simulink model "CM475A_TSG31CfgAndUse"  (R2013b)
settings: Solver=FixedStepDiscrete  SolverMode=SingleTasking  StartTime=0.0  StopTime=0.5  FixedStep=0.00005  RelTol=1e-3
undefined symbols (not defined in the file): ELECGLBPRM_PWMPERDMIN_NANOSEC_U32, sigbuilder_block, SysSt1, TSG31CfgAndUseAdcStrtOfCnvn2Offs, TSG31CfgAndUseAdcStrtOfCnvnMotCtrlPeakOffs, TSG31CfgAndUseAdcStrtOfCnvnMotCtrlVlyOffs, TSG31CfgAndUseMtrAg0SPIStart, TSG31CfgAndUsePwmDbnd, TSG31UPD_NANOSEC_U32
libraries: simulink x11, CM475A_TSG31CfgAndUse_ModelLibrary_Rev001 x11
(part 4 of 4)

== system CM475A_TSG31CfgAndUse/TSG31CfgAndUse/TSG31CfgAndUsePer2/No Transition SysState = Enable/MCECS_OFFSCMDEND and MCECS_GAINCMDAD/Map Pins to GPIO/IoHwAb_SetFctGpioPhaALowrCmd ==
  CopyRight2 : Subsystem  Description=|  mask(Copyright Information){none=on}
      | Copyright info block.                                               
      |                                                                     
      | Place copyright information at the top of every subsystem in design.
      mask prompts: none "No parameters"
      mask help: Place copyright information at the top of every subsystem in design.
      mask Display:
      | NxtrConf = 'Nexteer Confidential';
      | 
      | sys = bdroot; %handle for the current model ("system")
      | first = get_param(sys,'Created');
      | first = first(end-3:end);  %year is last four digits
      | 
      | last = get_param(sys,'LastModifiedDate');
      | if isempty(last)
      |     last = datestr(now,'yyyy');
      | else
      |     last = last(end-3:end);
      | end
      | 
      | if strcmp(first,last)
      |     fprintf('%s -- Copyright %s Nexteer',NxtrConf,first)
      | else
      |     fprintf('%s -- %s%s- %s Nexteer',NxtrConf,char(169),first,last)
      | end

== system CM475A_TSG31CfgAndUse/TSG31CfgAndUse/TSG31CfgAndUsePer2/No Transition SysState = Enable/MCECS_OFFSCMDEND and MCECS_GAINCMDAD/Map Pins to GPIO/IoHwAb_SetFctGpioPhaAUpprCmd ==
  CopyRight2 : Subsystem  Description=|  mask(Copyright Information){none=on}
      | Copyright info block.                                               
      |                                                                     
      | Place copyright information at the top of every subsystem in design.
      mask prompts: none "No parameters"
      mask help: Place copyright information at the top of every subsystem in design.
      mask Display:
      | NxtrConf = 'Nexteer Confidential';
      | 
      | sys = bdroot; %handle for the current model ("system")
      | first = get_param(sys,'Created');
      | first = first(end-3:end);  %year is last four digits
      | 
      | last = get_param(sys,'LastModifiedDate');
      | if isempty(last)
      |     last = datestr(now,'yyyy');
      | else
      |     last = last(end-3:end);
      | end
      | 
      | if strcmp(first,last)
      |     fprintf('%s -- Copyright %s Nexteer',NxtrConf,first)
      | else
      |     fprintf('%s -- %s%s- %s Nexteer',NxtrConf,char(169),first,last)
      | end

== system CM475A_TSG31CfgAndUse/TSG31CfgAndUse/TSG31CfgAndUsePer2/No Transition SysState = Enable/MCECS_OFFSCMDEND and MCECS_GAINCMDAD/Map Pins to GPIO/IoHwAb_SetFctGpioPhaBLowrCmd ==
  CopyRight2 : Subsystem  Description=|  mask(Copyright Information){none=on}
      | Copyright info block.                                               
      |                                                                     
      | Place copyright information at the top of every subsystem in design.
      mask prompts: none "No parameters"
      mask help: Place copyright information at the top of every subsystem in design.
      mask Display:
      | NxtrConf = 'Nexteer Confidential';
      | 
      | sys = bdroot; %handle for the current model ("system")
      | first = get_param(sys,'Created');
      | first = first(end-3:end);  %year is last four digits
      | 
      | last = get_param(sys,'LastModifiedDate');
      | if isempty(last)
      |     last = datestr(now,'yyyy');
      | else
      |     last = last(end-3:end);
      | end
      | 
      | if strcmp(first,last)
      |     fprintf('%s -- Copyright %s Nexteer',NxtrConf,first)
      | else
      |     fprintf('%s -- %s%s- %s Nexteer',NxtrConf,char(169),first,last)
      | end

== system CM475A_TSG31CfgAndUse/TSG31CfgAndUse/TSG31CfgAndUsePer2/No Transition SysState = Enable/MCECS_OFFSCMDEND and MCECS_GAINCMDAD/Map Pins to GPIO/IoHwAb_SetFctGpioPhaBUpprCmd ==
  CopyRight2 : Subsystem  Description=|  mask(Copyright Information){none=on}
      | Copyright info block.                                               
      |                                                                     
      | Place copyright information at the top of every subsystem in design.
      mask prompts: none "No parameters"
      mask help: Place copyright information at the top of every subsystem in design.
      mask Display:
      | NxtrConf = 'Nexteer Confidential';
      | 
      | sys = bdroot; %handle for the current model ("system")
      | first = get_param(sys,'Created');
      | first = first(end-3:end);  %year is last four digits
      | 
      | last = get_param(sys,'LastModifiedDate');
      | if isempty(last)
      |     last = datestr(now,'yyyy');
      | else
      |     last = last(end-3:end);
      | end
      | 
      | if strcmp(first,last)
      |     fprintf('%s -- Copyright %s Nexteer',NxtrConf,first)
      | else
      |     fprintf('%s -- %s%s- %s Nexteer',NxtrConf,char(169),first,last)
      | end

== system CM475A_TSG31CfgAndUse/TSG31CfgAndUse/TSG31CfgAndUsePer2/No Transition SysState = Enable/MCECS_OFFSCMDEND and MCECS_GAINCMDAD/Map Pins to GPIO/IoHwAb_SetFctGpioPhaCLowrCmd ==
  CopyRight2 : Subsystem  Description=|  mask(Copyright Information){none=on}
      | Copyright info block.                                               
      |                                                                     
      | Place copyright information at the top of every subsystem in design.
      mask prompts: none "No parameters"
      mask help: Place copyright information at the top of every subsystem in design.
      mask Display:
      | NxtrConf = 'Nexteer Confidential';
      | 
      | sys = bdroot; %handle for the current model ("system")
      | first = get_param(sys,'Created');
      | first = first(end-3:end);  %year is last four digits
      | 
      | last = get_param(sys,'LastModifiedDate');
      | if isempty(last)
      |     last = datestr(now,'yyyy');
      | else
      |     last = last(end-3:end);
      | end
      | 
      | if strcmp(first,last)
      |     fprintf('%s -- Copyright %s Nexteer',NxtrConf,first)
      | else
      |     fprintf('%s -- %s%s- %s Nexteer',NxtrConf,char(169),first,last)
      | end

== system CM475A_TSG31CfgAndUse/TSG31CfgAndUse/TSG31CfgAndUsePer2/No Transition SysState = Enable/MCECS_OFFSCMDEND and MCECS_GAINCMDAD/Map Pins to GPIO/IoHwAb_SetFctGpioPhaCUpprCmd ==
  CopyRight2 : Subsystem  Description=|  mask(Copyright Information){none=on}
      | Copyright info block.                                               
      |                                                                     
      | Place copyright information at the top of every subsystem in design.
      mask prompts: none "No parameters"
      mask help: Place copyright information at the top of every subsystem in design.
      mask Display:
      | NxtrConf = 'Nexteer Confidential';
      | 
      | sys = bdroot; %handle for the current model ("system")
      | first = get_param(sys,'Created');
      | first = first(end-3:end);  %year is last four digits
      | 
      | last = get_param(sys,'LastModifiedDate');
      | if isempty(last)
      |     last = datestr(now,'yyyy');
      | else
      |     last = last(end-3:end);
      | end
      | 
      | if strcmp(first,last)
      |     fprintf('%s -- Copyright %s Nexteer',NxtrConf,first)
      | else
      |     fprintf('%s -- %s%s- %s Nexteer',NxtrConf,char(169),first,last)
      | end

== system CM475A_TSG31CfgAndUse/TSG31CfgAndUse/TSG31CfgAndUsePer2/No Transition SysState = Enable/MCECS_OFFSCMDEND and MCECS_GAINCMDAD/Set GPIO Level/CopyRight2 ==

== system CM475A_TSG31CfgAndUse/TSG31CfgAndUse/TSG31CfgAndUsePer2/No Transition SysState = Enable/MCECS_OFFSCMDEND and MCECS_GAINCMDAD/Set GPIO Level/IoHwAb_SetGpioPhaALowrCmd ==
  PinSt : Inport  OutDataTypeStr=boolean
  CopyRight2 : Subsystem  Description=|  mask(Copyright Information){none=on}
      | Copyright info block.                                               
      |                                                                     
      | Place copyright information at the top of every subsystem in design.
      mask prompts: none "No parameters"
      mask help: Place copyright information at the top of every subsystem in design.
      mask Display:
      | NxtrConf = 'Nexteer Confidential';
      | 
      | sys = bdroot; %handle for the current model ("system")
      | first = get_param(sys,'Created');
      | first = first(end-3:end);  %year is last four digits
      | 
      | last = get_param(sys,'LastModifiedDate');
      | if isempty(last)
      |     last = datestr(now,'yyyy');
      | else
      |     last = last(end-3:end);
      | end
      | 
      | if strcmp(first,last)
      |     fprintf('%s -- Copyright %s Nexteer',NxtrConf,first)
      | else
      |     fprintf('%s -- %s%s- %s Nexteer',NxtrConf,char(169),first,last)
      | end
  Terminator : Terminator
  wires:
  PinSt/1 -> Terminator/1

== system CM475A_TSG31CfgAndUse/TSG31CfgAndUse/TSG31CfgAndUsePer2/No Transition SysState = Enable/MCECS_OFFSCMDEND and MCECS_GAINCMDAD/Set GPIO Level/IoHwAb_SetGpioPhaAUpprCmd ==
  PinSt : Inport  OutDataTypeStr=boolean
  CopyRight2 : Subsystem  Description=|  mask(Copyright Information){none=on}
      | Copyright info block.                                               
      |                                                                     
      | Place copyright information at the top of every subsystem in design.
      mask prompts: none "No parameters"
      mask help: Place copyright information at the top of every subsystem in design.
      mask Display:
      | NxtrConf = 'Nexteer Confidential';
      | 
      | sys = bdroot; %handle for the current model ("system")
      | first = get_param(sys,'Created');
      | first = first(end-3:end);  %year is last four digits
      | 
      | last = get_param(sys,'LastModifiedDate');
      | if isempty(last)
      |     last = datestr(now,'yyyy');
      | else
      |     last = last(end-3:end);
      | end
      | 
      | if strcmp(first,last)
      |     fprintf('%s -- Copyright %s Nexteer',NxtrConf,first)
      | else
      |     fprintf('%s -- %s%s- %s Nexteer',NxtrConf,char(169),first,last)
      | end
  Terminator : Terminator
  wires:
  PinSt/1 -> Terminator/1

== system CM475A_TSG31CfgAndUse/TSG31CfgAndUse/TSG31CfgAndUsePer2/No Transition SysState = Enable/MCECS_OFFSCMDEND and MCECS_GAINCMDAD/Set GPIO Level/IoHwAb_SetGpioPhaBLowrCmd ==
  PinSt : Inport  OutDataTypeStr=boolean
  CopyRight2 : Subsystem  Description=|  mask(Copyright Information){none=on}
      | Copyright info block.                                               
      |                                                                     
      | Place copyright information at the top of every subsystem in design.
      mask prompts: none "No parameters"
      mask help: Place copyright information at the top of every subsystem in design.
      mask Display:
      | NxtrConf = 'Nexteer Confidential';
      | 
      | sys = bdroot; %handle for the current model ("system")
      | first = get_param(sys,'Created');
      | first = first(end-3:end);  %year is last four digits
      | 
      | last = get_param(sys,'LastModifiedDate');
      | if isempty(last)
      |     last = datestr(now,'yyyy');
      | else
      |     last = last(end-3:end);
      | end
      | 
      | if strcmp(first,last)
      |     fprintf('%s -- Copyright %s Nexteer',NxtrConf,first)
      | else
      |     fprintf('%s -- %s%s- %s Nexteer',NxtrConf,char(169),first,last)
      | end
  Terminator : Terminator
  wires:
  PinSt/1 -> Terminator/1

== system CM475A_TSG31CfgAndUse/TSG31CfgAndUse/TSG31CfgAndUsePer2/No Transition SysState = Enable/MCECS_OFFSCMDEND and MCECS_GAINCMDAD/Set GPIO Level/IoHwAb_SetGpioPhaBUpprCmd ==
  PinSt : Inport  OutDataTypeStr=boolean
  CopyRight2 : Subsystem  Description=|  mask(Copyright Information){none=on}
      | Copyright info block.                                               
      |                                                                     
      | Place copyright information at the top of every subsystem in design.
      mask prompts: none "No parameters"
      mask help: Place copyright information at the top of every subsystem in design.
      mask Display:
      | NxtrConf = 'Nexteer Confidential';
      | 
      | sys = bdroot; %handle for the current model ("system")
      | first = get_param(sys,'Created');
      | first = first(end-3:end);  %year is last four digits
      | 
      | last = get_param(sys,'LastModifiedDate');
      | if isempty(last)
      |     last = datestr(now,'yyyy');
      | else
      |     last = last(end-3:end);
      | end
      | 
      | if strcmp(first,last)
      |     fprintf('%s -- Copyright %s Nexteer',NxtrConf,first)
      | else
      |     fprintf('%s -- %s%s- %s Nexteer',NxtrConf,char(169),first,last)
      | end
  Terminator : Terminator
  wires:
  PinSt/1 -> Terminator/1

== system CM475A_TSG31CfgAndUse/TSG31CfgAndUse/TSG31CfgAndUsePer2/No Transition SysState = Enable/MCECS_OFFSCMDEND and MCECS_GAINCMDAD/Set GPIO Level/IoHwAb_SetGpioPhaCLowrCmd ==
  PinSt : Inport  OutDataTypeStr=boolean
  CopyRight2 : Subsystem  Description=|  mask(Copyright Information){none=on}
      | Copyright info block.                                               
      |                                                                     
      | Place copyright information at the top of every subsystem in design.
      mask prompts: none "No parameters"
      mask help: Place copyright information at the top of every subsystem in design.
      mask Display:
      | NxtrConf = 'Nexteer Confidential';
      | 
      | sys = bdroot; %handle for the current model ("system")
      | first = get_param(sys,'Created');
      | first = first(end-3:end);  %year is last four digits
      | 
      | last = get_param(sys,'LastModifiedDate');
      | if isempty(last)
      |     last = datestr(now,'yyyy');
      | else
      |     last = last(end-3:end);
      | end
      | 
      | if strcmp(first,last)
      |     fprintf('%s -- Copyright %s Nexteer',NxtrConf,first)
      | else
      |     fprintf('%s -- %s%s- %s Nexteer',NxtrConf,char(169),first,last)
      | end
  Terminator : Terminator
  wires:
  PinSt/1 -> Terminator/1

== system CM475A_TSG31CfgAndUse/TSG31CfgAndUse/TSG31CfgAndUsePer2/No Transition SysState = Enable/MCECS_OFFSCMDEND and MCECS_GAINCMDAD/Set GPIO Level/IoHwAb_SetGpioPhaCUpprCmd ==
  PinSt : Inport  OutDataTypeStr=boolean
  CopyRight2 : Subsystem  Description=|  mask(Copyright Information){none=on}
      | Copyright info block.                                               
      |                                                                     
      | Place copyright information at the top of every subsystem in design.
      mask prompts: none "No parameters"
      mask help: Place copyright information at the top of every subsystem in design.
      mask Display:
      | NxtrConf = 'Nexteer Confidential';
      | 
      | sys = bdroot; %handle for the current model ("system")
      | first = get_param(sys,'Created');
      | first = first(end-3:end);  %year is last four digits
      | 
      | last = get_param(sys,'LastModifiedDate');
      | if isempty(last)
      |     last = datestr(now,'yyyy');
      | else
      |     last = last(end-3:end);
      | end
      | 
      | if strcmp(first,last)
      |     fprintf('%s -- Copyright %s Nexteer',NxtrConf,first)
      | else
      |     fprintf('%s -- %s%s- %s Nexteer',NxtrConf,char(169),first,last)
      | end
  Terminator : Terminator
  wires:
  PinSt/1 -> Terminator/1

== system CM475A_TSG31CfgAndUse/TSG31CfgAndUse/TSG31CfgAndUsePer2/Transition from Enable/Map FET Ctrl Signals to GPIO and Set Low/Map Pins to GPIO/CopyRight2 ==

== system CM475A_TSG31CfgAndUse/TSG31CfgAndUse/TSG31CfgAndUsePer2/Transition from Enable/Map FET Ctrl Signals to GPIO and Set Low/Map Pins to GPIO/IoHwAb_SetFctGpioPhaALowrCmd ==
  CopyRight2 : Subsystem  Description=|  mask(Copyright Information){none=on}
      | Copyright info block.                                               
      |                                                                     
      | Place copyright information at the top of every subsystem in design.
      mask prompts: none "No parameters"
      mask help: Place copyright information at the top of every subsystem in design.
      mask Display:
      | NxtrConf = 'Nexteer Confidential';
      | 
      | sys = bdroot; %handle for the current model ("system")
      | first = get_param(sys,'Created');
      | first = first(end-3:end);  %year is last four digits
      | 
      | last = get_param(sys,'LastModifiedDate');
      | if isempty(last)
      |     last = datestr(now,'yyyy');
      | else
      |     last = last(end-3:end);
      | end
      | 
      | if strcmp(first,last)
      |     fprintf('%s -- Copyright %s Nexteer',NxtrConf,first)
      | else
      |     fprintf('%s -- %s%s- %s Nexteer',NxtrConf,char(169),first,last)
      | end

== system CM475A_TSG31CfgAndUse/TSG31CfgAndUse/TSG31CfgAndUsePer2/Transition from Enable/Map FET Ctrl Signals to GPIO and Set Low/Map Pins to GPIO/IoHwAb_SetFctGpioPhaAUpprCmd ==
  CopyRight2 : Subsystem  Description=|  mask(Copyright Information){none=on}
      | Copyright info block.                                               
      |                                                                     
      | Place copyright information at the top of every subsystem in design.
      mask prompts: none "No parameters"
      mask help: Place copyright information at the top of every subsystem in design.
      mask Display:
      | NxtrConf = 'Nexteer Confidential';
      | 
      | sys = bdroot; %handle for the current model ("system")
      | first = get_param(sys,'Created');
      | first = first(end-3:end);  %year is last four digits
      | 
      | last = get_param(sys,'LastModifiedDate');
      | if isempty(last)
      |     last = datestr(now,'yyyy');
      | else
      |     last = last(end-3:end);
      | end
      | 
      | if strcmp(first,last)
      |     fprintf('%s -- Copyright %s Nexteer',NxtrConf,first)
      | else
      |     fprintf('%s -- %s%s- %s Nexteer',NxtrConf,char(169),first,last)
      | end

== system CM475A_TSG31CfgAndUse/TSG31CfgAndUse/TSG31CfgAndUsePer2/Transition from Enable/Map FET Ctrl Signals to GPIO and Set Low/Map Pins to GPIO/IoHwAb_SetFctGpioPhaBLowrCmd ==
  CopyRight2 : Subsystem  Description=|  mask(Copyright Information){none=on}
      | Copyright info block.                                               
      |                                                                     
      | Place copyright information at the top of every subsystem in design.
      mask prompts: none "No parameters"
      mask help: Place copyright information at the top of every subsystem in design.
      mask Display:
      | NxtrConf = 'Nexteer Confidential';
      | 
      | sys = bdroot; %handle for the current model ("system")
      | first = get_param(sys,'Created');
      | first = first(end-3:end);  %year is last four digits
      | 
      | last = get_param(sys,'LastModifiedDate');
      | if isempty(last)
      |     last = datestr(now,'yyyy');
      | else
      |     last = last(end-3:end);
      | end
      | 
      | if strcmp(first,last)
      |     fprintf('%s -- Copyright %s Nexteer',NxtrConf,first)
      | else
      |     fprintf('%s -- %s%s- %s Nexteer',NxtrConf,char(169),first,last)
      | end

== system CM475A_TSG31CfgAndUse/TSG31CfgAndUse/TSG31CfgAndUsePer2/Transition from Enable/Map FET Ctrl Signals to GPIO and Set Low/Map Pins to GPIO/IoHwAb_SetFctGpioPhaBUpprCmd ==
  CopyRight2 : Subsystem  Description=|  mask(Copyright Information){none=on}
      | Copyright info block.                                               
      |                                                                     
      | Place copyright information at the top of every subsystem in design.
      mask prompts: none "No parameters"
      mask help: Place copyright information at the top of every subsystem in design.
      mask Display:
      | NxtrConf = 'Nexteer Confidential';
      | 
      | sys = bdroot; %handle for the current model ("system")
      | first = get_param(sys,'Created');
      | first = first(end-3:end);  %year is last four digits
      | 
      | last = get_param(sys,'LastModifiedDate');
      | if isempty(last)
      |     last = datestr(now,'yyyy');
      | else
      |     last = last(end-3:end);
      | end
      | 
      | if strcmp(first,last)
      |     fprintf('%s -- Copyright %s Nexteer',NxtrConf,first)
      | else
      |     fprintf('%s -- %s%s- %s Nexteer',NxtrConf,char(169),first,last)
      | end

== system CM475A_TSG31CfgAndUse/TSG31CfgAndUse/TSG31CfgAndUsePer2/Transition from Enable/Map FET Ctrl Signals to GPIO and Set Low/Map Pins to GPIO/IoHwAb_SetFctGpioPhaCLowrCmd ==
  CopyRight2 : Subsystem  Description=|  mask(Copyright Information){none=on}
      | Copyright info block.                                               
      |                                                                     
      | Place copyright information at the top of every subsystem in design.
      mask prompts: none "No parameters"
      mask help: Place copyright information at the top of every subsystem in design.
      mask Display:
      | NxtrConf = 'Nexteer Confidential';
      | 
      | sys = bdroot; %handle for the current model ("system")
      | first = get_param(sys,'Created');
      | first = first(end-3:end);  %year is last four digits
      | 
      | last = get_param(sys,'LastModifiedDate');
      | if isempty(last)
      |     last = datestr(now,'yyyy');
      | else
      |     last = last(end-3:end);
      | end
      | 
      | if strcmp(first,last)
      |     fprintf('%s -- Copyright %s Nexteer',NxtrConf,first)
      | else
      |     fprintf('%s -- %s%s- %s Nexteer',NxtrConf,char(169),first,last)
      | end

== system CM475A_TSG31CfgAndUse/TSG31CfgAndUse/TSG31CfgAndUsePer2/Transition from Enable/Map FET Ctrl Signals to GPIO and Set Low/Map Pins to GPIO/IoHwAb_SetFctGpioPhaCUpprCmd ==
  CopyRight2 : Subsystem  Description=|  mask(Copyright Information){none=on}
      | Copyright info block.                                               
      |                                                                     
      | Place copyright information at the top of every subsystem in design.
      mask prompts: none "No parameters"
      mask help: Place copyright information at the top of every subsystem in design.
      mask Display:
      | NxtrConf = 'Nexteer Confidential';
      | 
      | sys = bdroot; %handle for the current model ("system")
      | first = get_param(sys,'Created');
      | first = first(end-3:end);  %year is last four digits
      | 
      | last = get_param(sys,'LastModifiedDate');
      | if isempty(last)
      |     last = datestr(now,'yyyy');
      | else
      |     last = last(end-3:end);
      | end
      | 
      | if strcmp(first,last)
      |     fprintf('%s -- Copyright %s Nexteer',NxtrConf,first)
      | else
      |     fprintf('%s -- %s%s- %s Nexteer',NxtrConf,char(169),first,last)
      | end

== system CM475A_TSG31CfgAndUse/TSG31CfgAndUse/TSG31CfgAndUsePer2/Transition from Enable/Map FET Ctrl Signals to GPIO and Set Low/Set GPIO Level/CopyRight2 ==

== system CM475A_TSG31CfgAndUse/TSG31CfgAndUse/TSG31CfgAndUsePer2/Transition from Enable/Map FET Ctrl Signals to GPIO and Set Low/Set GPIO Level/IoHwAb_SetGpioPhaALowrCmd ==
  PinSt : Inport  OutDataTypeStr=boolean
  CopyRight2 : Subsystem  Description=|  mask(Copyright Information){none=on}
      | Copyright info block.                                               
      |                                                                     
      | Place copyright information at the top of every subsystem in design.
      mask prompts: none "No parameters"
      mask help: Place copyright information at the top of every subsystem in design.
      mask Display:
      | NxtrConf = 'Nexteer Confidential';
      | 
      | sys = bdroot; %handle for the current model ("system")
      | first = get_param(sys,'Created');
      | first = first(end-3:end);  %year is last four digits
      | 
      | last = get_param(sys,'LastModifiedDate');
      | if isempty(last)
      |     last = datestr(now,'yyyy');
      | else
      |     last = last(end-3:end);
      | end
      | 
      | if strcmp(first,last)
      |     fprintf('%s -- Copyright %s Nexteer',NxtrConf,first)
      | else
      |     fprintf('%s -- %s%s- %s Nexteer',NxtrConf,char(169),first,last)
      | end
  Terminator : Terminator
  wires:
  PinSt/1 -> Terminator/1

== system CM475A_TSG31CfgAndUse/TSG31CfgAndUse/TSG31CfgAndUsePer2/Transition from Enable/Map FET Ctrl Signals to GPIO and Set Low/Set GPIO Level/IoHwAb_SetGpioPhaAUpprCmd ==
  PinSt : Inport  OutDataTypeStr=boolean
  CopyRight2 : Subsystem  Description=|  mask(Copyright Information){none=on}
      | Copyright info block.                                               
      |                                                                     
      | Place copyright information at the top of every subsystem in design.
      mask prompts: none "No parameters"
      mask help: Place copyright information at the top of every subsystem in design.
      mask Display:
      | NxtrConf = 'Nexteer Confidential';
      | 
      | sys = bdroot; %handle for the current model ("system")
      | first = get_param(sys,'Created');
      | first = first(end-3:end);  %year is last four digits
      | 
      | last = get_param(sys,'LastModifiedDate');
      | if isempty(last)
      |     last = datestr(now,'yyyy');
      | else
      |     last = last(end-3:end);
      | end
      | 
      | if strcmp(first,last)
      |     fprintf('%s -- Copyright %s Nexteer',NxtrConf,first)
      | else
      |     fprintf('%s -- %s%s- %s Nexteer',NxtrConf,char(169),first,last)
      | end
  Terminator : Terminator
  wires:
  PinSt/1 -> Terminator/1

== system CM475A_TSG31CfgAndUse/TSG31CfgAndUse/TSG31CfgAndUsePer2/Transition from Enable/Map FET Ctrl Signals to GPIO and Set Low/Set GPIO Level/IoHwAb_SetGpioPhaBLowrCmd ==
  PinSt : Inport  OutDataTypeStr=boolean
  CopyRight2 : Subsystem  Description=|  mask(Copyright Information){none=on}
      | Copyright info block.                                               
      |                                                                     
      | Place copyright information at the top of every subsystem in design.
      mask prompts: none "No parameters"
      mask help: Place copyright information at the top of every subsystem in design.
      mask Display:
      | NxtrConf = 'Nexteer Confidential';
      | 
      | sys = bdroot; %handle for the current model ("system")
      | first = get_param(sys,'Created');
      | first = first(end-3:end);  %year is last four digits
      | 
      | last = get_param(sys,'LastModifiedDate');
      | if isempty(last)
      |     last = datestr(now,'yyyy');
      | else
      |     last = last(end-3:end);
      | end
      | 
      | if strcmp(first,last)
      |     fprintf('%s -- Copyright %s Nexteer',NxtrConf,first)
      | else
      |     fprintf('%s -- %s%s- %s Nexteer',NxtrConf,char(169),first,last)
      | end
  Terminator : Terminator
  wires:
  PinSt/1 -> Terminator/1

== system CM475A_TSG31CfgAndUse/TSG31CfgAndUse/TSG31CfgAndUsePer2/Transition from Enable/Map FET Ctrl Signals to GPIO and Set Low/Set GPIO Level/IoHwAb_SetGpioPhaBUpprCmd ==
  PinSt : Inport  OutDataTypeStr=boolean
  CopyRight2 : Subsystem  Description=|  mask(Copyright Information){none=on}
      | Copyright info block.                                               
      |                                                                     
      | Place copyright information at the top of every subsystem in design.
      mask prompts: none "No parameters"
      mask help: Place copyright information at the top of every subsystem in design.
      mask Display:
      | NxtrConf = 'Nexteer Confidential';
      | 
      | sys = bdroot; %handle for the current model ("system")
      | first = get_param(sys,'Created');
      | first = first(end-3:end);  %year is last four digits
      | 
      | last = get_param(sys,'LastModifiedDate');
      | if isempty(last)
      |     last = datestr(now,'yyyy');
      | else
      |     last = last(end-3:end);
      | end
      | 
      | if strcmp(first,last)
      |     fprintf('%s -- Copyright %s Nexteer',NxtrConf,first)
      | else
      |     fprintf('%s -- %s%s- %s Nexteer',NxtrConf,char(169),first,last)
      | end
  Terminator : Terminator
  wires:
  PinSt/1 -> Terminator/1

== system CM475A_TSG31CfgAndUse/TSG31CfgAndUse/TSG31CfgAndUsePer2/Transition from Enable/Map FET Ctrl Signals to GPIO and Set Low/Set GPIO Level/IoHwAb_SetGpioPhaCLowrCmd ==
  PinSt : Inport  OutDataTypeStr=boolean
  CopyRight2 : Subsystem  Description=|  mask(Copyright Information){none=on}
      | Copyright info block.                                               
      |                                                                     
      | Place copyright information at the top of every subsystem in design.
      mask prompts: none "No parameters"
      mask help: Place copyright information at the top of every subsystem in design.
      mask Display:
      | NxtrConf = 'Nexteer Confidential';
      | 
      | sys = bdroot; %handle for the current model ("system")
      | first = get_param(sys,'Created');
      | first = first(end-3:end);  %year is last four digits
      | 
      | last = get_param(sys,'LastModifiedDate');
      | if isempty(last)
      |     last = datestr(now,'yyyy');
      | else
      |     last = last(end-3:end);
      | end
      | 
      | if strcmp(first,last)
      |     fprintf('%s -- Copyright %s Nexteer',NxtrConf,first)
      | else
      |     fprintf('%s -- %s%s- %s Nexteer',NxtrConf,char(169),first,last)
      | end
  Terminator : Terminator
  wires:
  PinSt/1 -> Terminator/1

== system CM475A_TSG31CfgAndUse/TSG31CfgAndUse/TSG31CfgAndUsePer2/Transition from Enable/Map FET Ctrl Signals to GPIO and Set Low/Set GPIO Level/IoHwAb_SetGpioPhaCUpprCmd ==
  PinSt : Inport  OutDataTypeStr=boolean
  CopyRight2 : Subsystem  Description=|  mask(Copyright Information){none=on}
      | Copyright info block.                                               
      |                                                                     
      | Place copyright information at the top of every subsystem in design.
      mask prompts: none "No parameters"
      mask help: Place copyright information at the top of every subsystem in design.
      mask Display:
      | NxtrConf = 'Nexteer Confidential';
      | 
      | sys = bdroot; %handle for the current model ("system")
      | first = get_param(sys,'Created');
      | first = first(end-3:end);  %year is last four digits
      | 
      | last = get_param(sys,'LastModifiedDate');
      | if isempty(last)
      |     last = datestr(now,'yyyy');
      | else
      |     last = last(end-3:end);
      | end
      | 
      | if strcmp(first,last)
      |     fprintf('%s -- Copyright %s Nexteer',NxtrConf,first)
      | else
      |     fprintf('%s -- %s%s- %s Nexteer',NxtrConf,char(169),first,last)
      | end
  Terminator : Terminator
  wires:
  PinSt/1 -> Terminator/1

== system CM475A_TSG31CfgAndUse/TSG31CfgAndUse/TSG31CfgAndUsePer2/Transition to Enable/Map Pins to Peripheral/IoHwAb_SetFctPeriphPhaALowrCmd/CopyRight2 ==

== system CM475A_TSG31CfgAndUse/TSG31CfgAndUse/TSG31CfgAndUsePer2/Transition to Enable/Map Pins to Peripheral/IoHwAb_SetFctPeriphPhaAUpprCmd/CopyRight2 ==

== system CM475A_TSG31CfgAndUse/TSG31CfgAndUse/TSG31CfgAndUsePer2/Transition to Enable/Map Pins to Peripheral/IoHwAb_SetFctPeriphPhaBLowrCmd/CopyRight2 ==

== system CM475A_TSG31CfgAndUse/TSG31CfgAndUse/TSG31CfgAndUsePer2/Transition to Enable/Map Pins to Peripheral/IoHwAb_SetFctPeriphPhaBUpprCmd/CopyRight2 ==

== system CM475A_TSG31CfgAndUse/TSG31CfgAndUse/TSG31CfgAndUsePer2/Transition to Enable/Map Pins to Peripheral/IoHwAb_SetFctPeriphPhaCLowrCmd/CopyRight2 ==

== system CM475A_TSG31CfgAndUse/TSG31CfgAndUse/TSG31CfgAndUsePer2/Transition to Enable/Map Pins to Peripheral/IoHwAb_SetFctPeriphPhaCUpprCmd/CopyRight2 ==

== system CM475A_TSG31CfgAndUse/TSG31CfgAndUse/TSG31CfgAndUsePer2/No Transition SysState = Enable/MCECS_CMDSAFEST/Map Pins to GPIO/IoHwAb_SetFctGpioPhaALowrCmd/CopyRight2 ==

== system CM475A_TSG31CfgAndUse/TSG31CfgAndUse/TSG31CfgAndUsePer2/No Transition SysState = Enable/MCECS_CMDSAFEST/Map Pins to GPIO/IoHwAb_SetFctGpioPhaAUpprCmd/CopyRight2 ==

== system CM475A_TSG31CfgAndUse/TSG31CfgAndUse/TSG31CfgAndUsePer2/No Transition SysState = Enable/MCECS_CMDSAFEST/Map Pins to GPIO/IoHwAb_SetFctGpioPhaBLowrCmd/CopyRight2 ==

== system CM475A_TSG31CfgAndUse/TSG31CfgAndUse/TSG31CfgAndUsePer2/No Transition SysState = Enable/MCECS_CMDSAFEST/Map Pins to GPIO/IoHwAb_SetFctGpioPhaBUpprCmd/CopyRight2 ==

== system CM475A_TSG31CfgAndUse/TSG31CfgAndUse/TSG31CfgAndUsePer2/No Transition SysState = Enable/MCECS_CMDSAFEST/Map Pins to GPIO/IoHwAb_SetFctGpioPhaCLowrCmd/CopyRight2 ==

== system CM475A_TSG31CfgAndUse/TSG31CfgAndUse/TSG31CfgAndUsePer2/No Transition SysState = Enable/MCECS_CMDSAFEST/Map Pins to GPIO/IoHwAb_SetFctGpioPhaCUpprCmd/CopyRight2 ==

== system CM475A_TSG31CfgAndUse/TSG31CfgAndUse/TSG31CfgAndUsePer2/No Transition SysState = Enable/MCECS_CMDSAFEST/Set GPIO Level/IoHwAb_SetGpioPhaALowrCmd/CopyRight2 ==

== system CM475A_TSG31CfgAndUse/TSG31CfgAndUse/TSG31CfgAndUsePer2/No Transition SysState = Enable/MCECS_CMDSAFEST/Set GPIO Level/IoHwAb_SetGpioPhaAUpprCmd/CopyRight2 ==

== system CM475A_TSG31CfgAndUse/TSG31CfgAndUse/TSG31CfgAndUsePer2/No Transition SysState = Enable/MCECS_CMDSAFEST/Set GPIO Level/IoHwAb_SetGpioPhaBLowrCmd/CopyRight2 ==

== system CM475A_TSG31CfgAndUse/TSG31CfgAndUse/TSG31CfgAndUsePer2/No Transition SysState = Enable/MCECS_CMDSAFEST/Set GPIO Level/IoHwAb_SetGpioPhaBUpprCmd/CopyRight2 ==

== system CM475A_TSG31CfgAndUse/TSG31CfgAndUse/TSG31CfgAndUsePer2/No Transition SysState = Enable/MCECS_CMDSAFEST/Set GPIO Level/IoHwAb_SetGpioPhaCLowrCmd/CopyRight2 ==

== system CM475A_TSG31CfgAndUse/TSG31CfgAndUse/TSG31CfgAndUsePer2/No Transition SysState = Enable/MCECS_CMDSAFEST/Set GPIO Level/IoHwAb_SetGpioPhaCUpprCmd/CopyRight2 ==

== system CM475A_TSG31CfgAndUse/TSG31CfgAndUse/TSG31CfgAndUsePer2/No Transition SysState = Enable/MCECS_GAINCMDBE/Map Pins to GPIO/IoHwAb_SetFctGpioPhaALowrCmd/CopyRight2 ==

== system CM475A_TSG31CfgAndUse/TSG31CfgAndUse/TSG31CfgAndUsePer2/No Transition SysState = Enable/MCECS_GAINCMDBE/Map Pins to GPIO/IoHwAb_SetFctGpioPhaAUpprCmd/CopyRight2 ==

== system CM475A_TSG31CfgAndUse/TSG31CfgAndUse/TSG31CfgAndUsePer2/No Transition SysState = Enable/MCECS_GAINCMDBE/Map Pins to GPIO/IoHwAb_SetFctGpioPhaBLowrCmd/CopyRight2 ==

== system CM475A_TSG31CfgAndUse/TSG31CfgAndUse/TSG31CfgAndUsePer2/No Transition SysState = Enable/MCECS_GAINCMDBE/Map Pins to GPIO/IoHwAb_SetFctGpioPhaBUpprCmd/CopyRight2 ==

== system CM475A_TSG31CfgAndUse/TSG31CfgAndUse/TSG31CfgAndUsePer2/No Transition SysState = Enable/MCECS_GAINCMDBE/Map Pins to GPIO/IoHwAb_SetFctGpioPhaCLowrCmd/CopyRight2 ==

== system CM475A_TSG31CfgAndUse/TSG31CfgAndUse/TSG31CfgAndUsePer2/No Transition SysState = Enable/MCECS_GAINCMDBE/Map Pins to GPIO/IoHwAb_SetFctGpioPhaCUpprCmd/CopyRight2 ==

== system CM475A_TSG31CfgAndUse/TSG31CfgAndUse/TSG31CfgAndUsePer2/No Transition SysState = Enable/MCECS_GAINCMDBE/Set GPIO Level/IoHwAb_SetGpioPhaALowrCmd/CopyRight2 ==

== system CM475A_TSG31CfgAndUse/TSG31CfgAndUse/TSG31CfgAndUsePer2/No Transition SysState = Enable/MCECS_GAINCMDBE/Set GPIO Level/IoHwAb_SetGpioPhaAUpprCmd/CopyRight2 ==

== system CM475A_TSG31CfgAndUse/TSG31CfgAndUse/TSG31CfgAndUsePer2/No Transition SysState = Enable/MCECS_GAINCMDBE/Set GPIO Level/IoHwAb_SetGpioPhaBLowrCmd/CopyRight2 ==

== system CM475A_TSG31CfgAndUse/TSG31CfgAndUse/TSG31CfgAndUsePer2/No Transition SysState = Enable/MCECS_GAINCMDBE/Set GPIO Level/IoHwAb_SetGpioPhaBUpprCmd/CopyRight2 ==

== system CM475A_TSG31CfgAndUse/TSG31CfgAndUse/TSG31CfgAndUsePer2/No Transition SysState = Enable/MCECS_GAINCMDBE/Set GPIO Level/IoHwAb_SetGpioPhaCLowrCmd/CopyRight2 ==

== system CM475A_TSG31CfgAndUse/TSG31CfgAndUse/TSG31CfgAndUsePer2/No Transition SysState = Enable/MCECS_GAINCMDBE/Set GPIO Level/IoHwAb_SetGpioPhaCUpprCmd/CopyRight2 ==

== system CM475A_TSG31CfgAndUse/TSG31CfgAndUse/TSG31CfgAndUsePer2/No Transition SysState = Enable/MCECS_GAINCMDCF/Map Pins to GPIO/IoHwAb_SetFctGpioPhaALowrCmd/CopyRight2 ==

== system CM475A_TSG31CfgAndUse/TSG31CfgAndUse/TSG31CfgAndUsePer2/No Transition SysState = Enable/MCECS_GAINCMDCF/Map Pins to GPIO/IoHwAb_SetFctGpioPhaAUpprCmd/CopyRight2 ==

== system CM475A_TSG31CfgAndUse/TSG31CfgAndUse/TSG31CfgAndUsePer2/No Transition SysState = Enable/MCECS_GAINCMDCF/Map Pins to GPIO/IoHwAb_SetFctGpioPhaBLowrCmd/CopyRight2 ==

== system CM475A_TSG31CfgAndUse/TSG31CfgAndUse/TSG31CfgAndUsePer2/No Transition SysState = Enable/MCECS_GAINCMDCF/Map Pins to GPIO/IoHwAb_SetFctGpioPhaBUpprCmd/CopyRight2 ==

== system CM475A_TSG31CfgAndUse/TSG31CfgAndUse/TSG31CfgAndUsePer2/No Transition SysState = Enable/MCECS_GAINCMDCF/Map Pins to GPIO/IoHwAb_SetFctGpioPhaCLowrCmd/CopyRight2 ==

== system CM475A_TSG31CfgAndUse/TSG31CfgAndUse/TSG31CfgAndUsePer2/No Transition SysState = Enable/MCECS_GAINCMDCF/Map Pins to GPIO/IoHwAb_SetFctGpioPhaCUpprCmd/CopyRight2 ==

== system CM475A_TSG31CfgAndUse/TSG31CfgAndUse/TSG31CfgAndUsePer2/No Transition SysState = Enable/MCECS_GAINCMDCF/Set GPIO Level/IoHwAb_SetGpioPhaALowrCmd/CopyRight2 ==

== system CM475A_TSG31CfgAndUse/TSG31CfgAndUse/TSG31CfgAndUsePer2/No Transition SysState = Enable/MCECS_GAINCMDCF/Set GPIO Level/IoHwAb_SetGpioPhaAUpprCmd/CopyRight2 ==

== system CM475A_TSG31CfgAndUse/TSG31CfgAndUse/TSG31CfgAndUsePer2/No Transition SysState = Enable/MCECS_GAINCMDCF/Set GPIO Level/IoHwAb_SetGpioPhaBLowrCmd/CopyRight2 ==

== system CM475A_TSG31CfgAndUse/TSG31CfgAndUse/TSG31CfgAndUsePer2/No Transition SysState = Enable/MCECS_GAINCMDCF/Set GPIO Level/IoHwAb_SetGpioPhaBUpprCmd/CopyRight2 ==

== system CM475A_TSG31CfgAndUse/TSG31CfgAndUse/TSG31CfgAndUsePer2/No Transition SysState = Enable/MCECS_GAINCMDCF/Set GPIO Level/IoHwAb_SetGpioPhaCLowrCmd/CopyRight2 ==

== system CM475A_TSG31CfgAndUse/TSG31CfgAndUse/TSG31CfgAndUsePer2/No Transition SysState = Enable/MCECS_GAINCMDCF/Set GPIO Level/IoHwAb_SetGpioPhaCUpprCmd/CopyRight2 ==

== system CM475A_TSG31CfgAndUse/TSG31CfgAndUse/TSG31CfgAndUsePer2/No Transition SysState = Enable/MCECS_OFFSCMDEND and MCECS_GAINCMDAD/Map Pins to GPIO/IoHwAb_SetFctGpioPhaALowrCmd/CopyRight2 ==

== system CM475A_TSG31CfgAndUse/TSG31CfgAndUse/TSG31CfgAndUsePer2/No Transition SysState = Enable/MCECS_OFFSCMDEND and MCECS_GAINCMDAD/Map Pins to GPIO/IoHwAb_SetFctGpioPhaAUpprCmd/CopyRight2 ==

== system CM475A_TSG31CfgAndUse/TSG31CfgAndUse/TSG31CfgAndUsePer2/No Transition SysState = Enable/MCECS_OFFSCMDEND and MCECS_GAINCMDAD/Map Pins to GPIO/IoHwAb_SetFctGpioPhaBLowrCmd/CopyRight2 ==

== system CM475A_TSG31CfgAndUse/TSG31CfgAndUse/TSG31CfgAndUsePer2/No Transition SysState = Enable/MCECS_OFFSCMDEND and MCECS_GAINCMDAD/Map Pins to GPIO/IoHwAb_SetFctGpioPhaBUpprCmd/CopyRight2 ==

== system CM475A_TSG31CfgAndUse/TSG31CfgAndUse/TSG31CfgAndUsePer2/No Transition SysState = Enable/MCECS_OFFSCMDEND and MCECS_GAINCMDAD/Map Pins to GPIO/IoHwAb_SetFctGpioPhaCLowrCmd/CopyRight2 ==

== system CM475A_TSG31CfgAndUse/TSG31CfgAndUse/TSG31CfgAndUsePer2/No Transition SysState = Enable/MCECS_OFFSCMDEND and MCECS_GAINCMDAD/Map Pins to GPIO/IoHwAb_SetFctGpioPhaCUpprCmd/CopyRight2 ==

== system CM475A_TSG31CfgAndUse/TSG31CfgAndUse/TSG31CfgAndUsePer2/No Transition SysState = Enable/MCECS_OFFSCMDEND and MCECS_GAINCMDAD/Set GPIO Level/IoHwAb_SetGpioPhaALowrCmd/CopyRight2 ==

== system CM475A_TSG31CfgAndUse/TSG31CfgAndUse/TSG31CfgAndUsePer2/No Transition SysState = Enable/MCECS_OFFSCMDEND and MCECS_GAINCMDAD/Set GPIO Level/IoHwAb_SetGpioPhaAUpprCmd/CopyRight2 ==

== system CM475A_TSG31CfgAndUse/TSG31CfgAndUse/TSG31CfgAndUsePer2/No Transition SysState = Enable/MCECS_OFFSCMDEND and MCECS_GAINCMDAD/Set GPIO Level/IoHwAb_SetGpioPhaBLowrCmd/CopyRight2 ==

== system CM475A_TSG31CfgAndUse/TSG31CfgAndUse/TSG31CfgAndUsePer2/No Transition SysState = Enable/MCECS_OFFSCMDEND and MCECS_GAINCMDAD/Set GPIO Level/IoHwAb_SetGpioPhaBUpprCmd/CopyRight2 ==

== system CM475A_TSG31CfgAndUse/TSG31CfgAndUse/TSG31CfgAndUsePer2/No Transition SysState = Enable/MCECS_OFFSCMDEND and MCECS_GAINCMDAD/Set GPIO Level/IoHwAb_SetGpioPhaCLowrCmd/CopyRight2 ==

== system CM475A_TSG31CfgAndUse/TSG31CfgAndUse/TSG31CfgAndUsePer2/No Transition SysState = Enable/MCECS_OFFSCMDEND and MCECS_GAINCMDAD/Set GPIO Level/IoHwAb_SetGpioPhaCUpprCmd/CopyRight2 ==

== system CM475A_TSG31CfgAndUse/TSG31CfgAndUse/TSG31CfgAndUsePer2/Transition from Enable/Map FET Ctrl Signals to GPIO and Set Low/Map Pins to GPIO/IoHwAb_SetFctGpioPhaALowrCmd/CopyRight2 ==

== system CM475A_TSG31CfgAndUse/TSG31CfgAndUse/TSG31CfgAndUsePer2/Transition from Enable/Map FET Ctrl Signals to GPIO and Set Low/Map Pins to GPIO/IoHwAb_SetFctGpioPhaAUpprCmd/CopyRight2 ==

== system CM475A_TSG31CfgAndUse/TSG31CfgAndUse/TSG31CfgAndUsePer2/Transition from Enable/Map FET Ctrl Signals to GPIO and Set Low/Map Pins to GPIO/IoHwAb_SetFctGpioPhaBLowrCmd/CopyRight2 ==

== system CM475A_TSG31CfgAndUse/TSG31CfgAndUse/TSG31CfgAndUsePer2/Transition from Enable/Map FET Ctrl Signals to GPIO and Set Low/Map Pins to GPIO/IoHwAb_SetFctGpioPhaBUpprCmd/CopyRight2 ==

== system CM475A_TSG31CfgAndUse/TSG31CfgAndUse/TSG31CfgAndUsePer2/Transition from Enable/Map FET Ctrl Signals to GPIO and Set Low/Map Pins to GPIO/IoHwAb_SetFctGpioPhaCLowrCmd/CopyRight2 ==

== system CM475A_TSG31CfgAndUse/TSG31CfgAndUse/TSG31CfgAndUsePer2/Transition from Enable/Map FET Ctrl Signals to GPIO and Set Low/Map Pins to GPIO/IoHwAb_SetFctGpioPhaCUpprCmd/CopyRight2 ==

== system CM475A_TSG31CfgAndUse/TSG31CfgAndUse/TSG31CfgAndUsePer2/Transition from Enable/Map FET Ctrl Signals to GPIO and Set Low/Set GPIO Level/IoHwAb_SetGpioPhaALowrCmd/CopyRight2 ==

== system CM475A_TSG31CfgAndUse/TSG31CfgAndUse/TSG31CfgAndUsePer2/Transition from Enable/Map FET Ctrl Signals to GPIO and Set Low/Set GPIO Level/IoHwAb_SetGpioPhaAUpprCmd/CopyRight2 ==

== system CM475A_TSG31CfgAndUse/TSG31CfgAndUse/TSG31CfgAndUsePer2/Transition from Enable/Map FET Ctrl Signals to GPIO and Set Low/Set GPIO Level/IoHwAb_SetGpioPhaBLowrCmd/CopyRight2 ==

== system CM475A_TSG31CfgAndUse/TSG31CfgAndUse/TSG31CfgAndUsePer2/Transition from Enable/Map FET Ctrl Signals to GPIO and Set Low/Set GPIO Level/IoHwAb_SetGpioPhaBUpprCmd/CopyRight2 ==

== system CM475A_TSG31CfgAndUse/TSG31CfgAndUse/TSG31CfgAndUsePer2/Transition from Enable/Map FET Ctrl Signals to GPIO and Set Low/Set GPIO Level/IoHwAb_SetGpioPhaCLowrCmd/CopyRight2 ==

== system CM475A_TSG31CfgAndUse/TSG31CfgAndUse/TSG31CfgAndUsePer2/Transition from Enable/Map FET Ctrl Signals to GPIO and Set Low/Set GPIO Level/IoHwAb_SetGpioPhaCUpprCmd/CopyRight2 ==

== matlab function CM475A_TSG31CfgAndUse/TSG31CfgAndUse/TSG31CfgAndUsePer2/Truth Table ==
  data: SysStateEnable input boolean; Out1 output; PrevSysStateEnable input boolean
function Out1 = fcn(SysStateEnable, PrevSysStateEnable)

aVarTruthTableCondition_1 = false;
aVarTruthTableCondition_2 = false;


% SysState = Enable

aVarTruthTableCondition_1 = logical(SysStateEnable == 1);

% PrevSysState = Enable

aVarTruthTableCondition_2 = logical(PrevSysStateEnable == 1);

if (aVarTruthTableCondition_1 && aVarTruthTableCondition_2)
    aFcnTruthTableAction_1();
elseif (~aVarTruthTableCondition_1 && aVarTruthTableCondition_2)
    aFcnTruthTableAction_2();
elseif (aVarTruthTableCondition_1 && ~aVarTruthTableCondition_2)
    aFcnTruthTableAction_3();
else % Default
    aFcnTruthTableAction_4();
end

function aFcnTruthTableAction_1()

% No Transition
% SysState = Enable

Out1 = 1;

function aFcnTruthTableAction_2()

% Transition from Enable

Out1 = 2;

function aFcnTruthTableAction_3()

% Transition to Enable

Out1 = 3;

function aFcnTruthTableAction_4()

% No Transition
% SysState != Enable

Out1 = 4;
